simulink model "under_actuated"  (R2020b)
settings: Solver=ode45  StartTime=0.0  StopTime=300  RelTol=1e-3
libraries: simulink x1
settings Model: Creator=kp473  LastModifiedBy=kp473
settings SolverCC: MaxConsecutiveMinStep=10

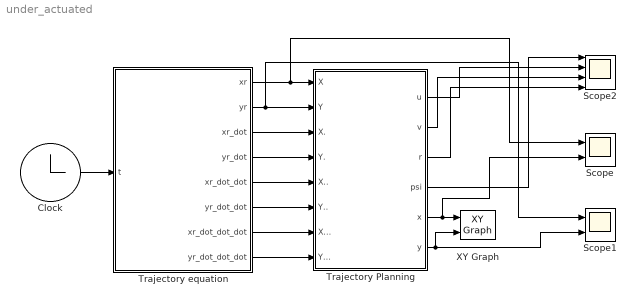
== system under_actuated ==
  Clock : Clock
      settings: Decimation=30
  Scope : Scope  NumInputPorts=2
  Scope1 : Scope  NumInputPorts=2
  Scope2 : Scope  NumInputPorts=4
  Trajectory Planning : Subsystem
  Trajectory equation : MATLAB Function  TreatAsAtomicUnit=on
  XY Graph : simulink/Sinks/XY Graph  xmin=-20  xmax=20  ymin=-20  ymax=20  st=-1
  wires:
  Clock/1 -> Trajectory equation/1(t)
  Trajectory equation/1(xr) -> Scope/1, Trajectory Planning/1(X)
  Trajectory equation/3(xr_dot) -> Trajectory Planning/3(X.)
  Trajectory equation/5(xr_dot_dot) -> Trajectory Planning/5(X..)
  Trajectory equation/2(yr) -> Scope1/1, Trajectory Planning/2(Y)
  Trajectory equation/4(yr_dot) -> Trajectory Planning/4(Y.)
  Trajectory equation/6(yr_dot_dot) -> Trajectory Planning/6(Y..)
  Trajectory equation/7(xr_dot_dot_dot) -> Trajectory Planning/7(X...)
  Trajectory equation/8(yr_dot_dot_dot) -> Trajectory Planning/8(Y...)
  Trajectory Planning/5(x) -> Scope/2, XY Graph/1
  Trajectory Planning/6(y) -> Scope1/2, XY Graph/2
  Trajectory Planning/4(psi) -> Scope2/1
  Trajectory Planning/1(u) -> Scope2/2
  Trajectory Planning/2(v) -> Scope2/3
  Trajectory Planning/3(r) -> Scope2/4

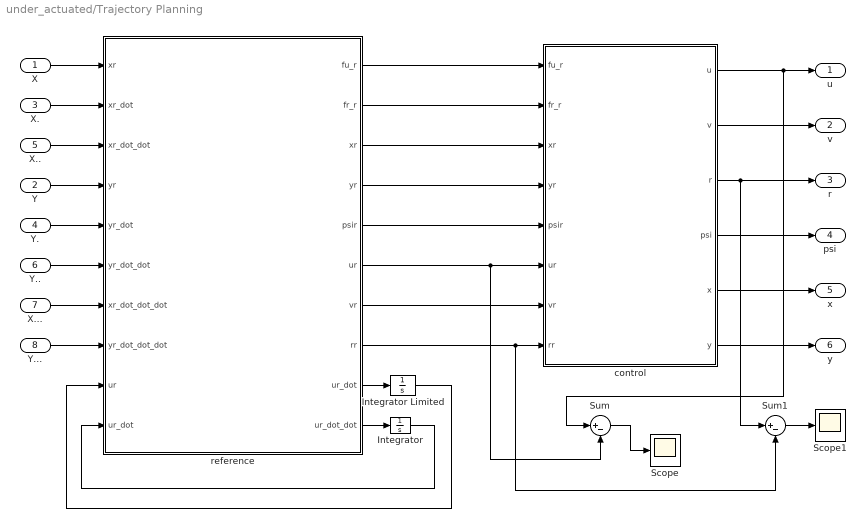
== system under_actuated/Trajectory Planning ==
  X : Inport
  Y : Inport  Port=2
  X. : Inport  Port=3
  Y. : Inport  Port=4
  X.. : Inport  Port=5
  Y.. : Inport  Port=6
  X... : Inport  Port=7
  Y... : Inport  Port=8
  Integrator : Integrator
  Integrator Limited : Integrator  InitialCondition=0.001  LimitOutput=on  UpperSaturationLimit=10  LowerSaturationLimit=-10
  Scope : Scope
  Scope1 : Scope
  Sum : Sum  Inputs=|+-
  Sum1 : Sum  Inputs=|+-
  control : Subsystem
  "reference " : MATLAB Function  TreatAsAtomicUnit=on
  u : Outport
  v : Outport  Port=2
  r : Outport  Port=3
  psi : Outport  Port=4
  x : Outport  Port=5
  y : Outport  Port=6
  wires:
  Y./1 -> "reference "/5(yr_dot)
  X/1 -> "reference "/1("xr ")
  Y../1 -> "reference "/6(yr_dot_dot)
  Y/1 -> "reference "/4("yr ")
  X./1 -> "reference "/2(xr_dot)
  X../1 -> "reference "/3(xr_dot_dot)
  X.../1 -> "reference "/7(xr_dot_dot_dot)
  Y.../1 -> "reference "/8(yr_dot_dot_dot)
  "reference "/10(ur_dot_dot) -> Integrator/1
  Integrator/1 -> "reference "/10("ur_dot ")
  "reference "/9(ur_dot) -> Integrator Limited/1
  Integrator Limited/1 -> "reference "/9("ur ")
  "reference "/1(fu_r) -> control/1(fu_r)
  "reference "/2(fr_r) -> control/2(fr_r)
  "reference "/3(xr) -> control/3(xr)
  "reference "/4(yr) -> control/4(yr)
  "reference "/5(psir) -> control/5(psir)
  "reference "/6(ur) -> Sum/2, control/6(ur)
  "reference "/7(vr) -> control/7(vr)
  "reference "/8(rr) -> Sum1/2, control/8(rr)
  control/1(u) -> Sum/1, u/1
  control/2(v) -> v/1
  control/3(r) -> Sum1/1, r/1
  control/4(psi) -> psi/1
  control/5(x) -> x/1
  control/6(y) -> y/1
  Sum/1 -> Scope/1
  Sum1/1 -> Scope1/1

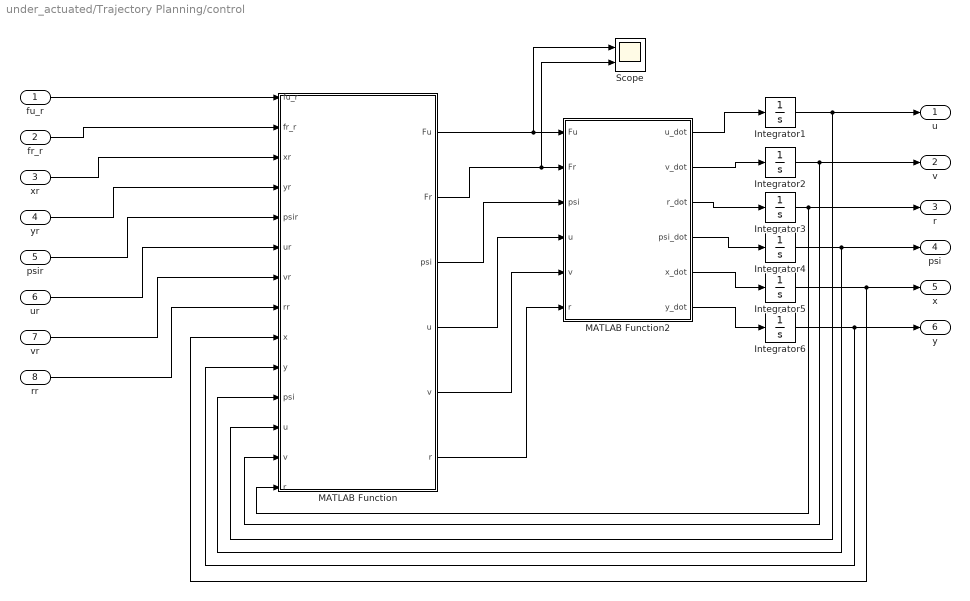
== system under_actuated/Trajectory Planning/control ==
  fu_r : Inport
  fr_r : Inport  Port=2
  xr : Inport  Port=3
  yr : Inport  Port=4
  psir : Inport  Port=5
  ur : Inport  Port=6
  vr : Inport  Port=7
  rr : Inport  Port=8
  Integrator{1..6} (6 alike) : Integrator
  MATLAB Function : MATLAB Function  TreatAsAtomicUnit=on
  MATLAB Function2 : MATLAB Function  TreatAsAtomicUnit=on
  Scope : Scope  NumInputPorts=2
  u : Outport
  v : Outport  Port=2
  r : Outport  Port=3
  psi : Outport  Port=4
  x : Outport  Port=5
  y : Outport  Port=6
  wires:
  Integrator2/1 -> v/1, MATLAB Function/13("v ")
  Integrator3/1 -> r/1, MATLAB Function/14("r ")
  rr/1 -> MATLAB Function/8(rr)
  MATLAB Function/4(u) -> MATLAB Function2/4(u)
  MATLAB Function2/1(u_dot) -> Integrator1/1
  MATLAB Function/2(Fr) -> Scope/2, MATLAB Function2/2(Fr)
  MATLAB Function2/5(x_dot) -> Integrator5/1
  MATLAB Function2/3(r_dot) -> Integrator3/1
  MATLAB Function/6(r) -> MATLAB Function2/6(r)
  Integrator1/1 -> u/1, MATLAB Function/12("u ")
  xr/1 -> MATLAB Function/3(xr)
  MATLAB Function2/2(v_dot) -> Integrator2/1
  Integrator6/1 -> y/1, MATLAB Function/10(y)
  MATLAB Function2/4(psi_dot) -> Integrator4/1
  yr/1 -> MATLAB Function/4(yr)
  Integrator4/1 -> psi/1, MATLAB Function/11("psi ")
  psir/1 -> MATLAB Function/5(psir)
  MATLAB Function/3(psi) -> MATLAB Function2/3(psi)
  MATLAB Function/5(v) -> MATLAB Function2/5(v)
  MATLAB Function/1(Fu) -> Scope/1, MATLAB Function2/1(Fu)
  MATLAB Function2/6(y_dot) -> Integrator6/1
  Integrator5/1 -> x/1, MATLAB Function/9(x)
  fu_r/1 -> MATLAB Function/1(fu_r)
  vr/1 -> MATLAB Function/7(vr)
  fr_r/1 -> MATLAB Function/2(fr_r)
  ur/1 -> MATLAB Function/6(ur)

== matlab function under_actuated/Trajectory equation ==
  data: xr output; yr output; t input; xr_dot output; yr_dot output; xr_dot_dot output; yr_dot_dot output; xr_dot_dot_dot output; yr_dot_dot_dot output
function [xr,yr,xr_dot,yr_dot,xr_dot_dot,yr_dot_dot,xr_dot_dot_dot,yr_dot_dot_dot] = fcn(t)

A = 10;
w = 0.1;

xr = A*sin(w*t);
yr = A*cos(w*t);

xr_dot = A*w*cos(w*t);
yr_dot = -A*w*sin(w*t);

xr_dot_dot = -A*w*w*sin(w*t);
yr_dot_dot = -A*w*w*cos(w*t);

xr_dot_dot_dot= -A*w*w*w*cos(w*t);
yr_dot_dot_dot= A*w*w*w*sin(w*t);

end

== matlab function under_actuated/Trajectory Planning/control/MATLAB Function ==
  data: fu_r input; Fu output; Fr output; fr_r input; xr input; yr input; psir input; ur input; vr input; rr input; x input; y input; psi input; u input; v input; r input; psi output; u output; v output; r output
function [Fu,Fr,psi,u,v,r] = fcn(fu_r, fr_r, xr, yr, psir, ur, vr, rr, x, y, psi, u, v, r)

% constants 
m= 185.0;                                                   % Mass kg
Iz = 50.0;                                                  % Moment of intertia
Xu = -30.0;                                                 
Yv = -90.0;                                                 
Nr = -30.0;                                                 
M = [(m-Xu); (m-Yv); (Iz-Nr)];                              % combined inertia and added mass terms
Minv = [1.0/(m-Xu); 1.0/(m-Yv); 1.0/(Iz-Nr)];               % one by combined inertia and added mass terms
dl = [70.0; 100.0; 50.0];  

% gain and errors
    e_xy = [ x - xr; y - yr];
    e_u = u - ur;
    e_v = v - vr;
    e_r = r - rr;
    e_psi = psi - psir;
    
    R = [ cos(psi), -sin(psi);
            sin(psi), cos(psi)];
    
    cu = 0.5;
    cr = 0.4;
    c = 0.6;
    kc = 0.2;
    
    k = 0.5;
    K = [k, 0;
        0, k];
    
    ku = 0.7;
    k1 = 0.7;
    K1 = [k1, 0;
        0, k1];
       
    alpha_uv = - transpose(R)*(K+K1)*e_xy;
    Zu = e_u - alpha_uv(1);
    Zv = e_v - alpha_uv(2);
    alpha_r = -cr*(-u*Zv*M(1)*Minv(2) + e_psi);
    Zr = e_r - alpha_r;
    
    
% Backstepping Control 
    T_u = -(k+k1)*e_u - cu*Zu - ku*Zu*(k+k1)*(k+k1);    
    T_r = -Zv - e_psi - cr*e_r*(((M(1)*u*Minv(2))^2)+1) - Zr*(c + kc*((cr*M(1)*u*Minv(2))^2));
    
% Updating Input of AUV ( Force and Torque )
    Fu = fu_r + M(1)*T_u + (dl(1)*e_u) - M(2)*(e_v*e_r + e_v*rr + vr*e_r);      
    Fr = fr_r + M(3)*T_r + (dl(3)*e_r) + (M(2)-M(1))*(e_u*e_v+ e_u*vr + ur*e_v);
    
end

== matlab function under_actuated/Trajectory Planning/reference  ==
  data: xr input; xr_dot input; xr_dot_dot input; fu_r output; yr input; yr_dot input; yr_dot_dot input; xr_dot_dot_dot input; yr_dot_dot_dot input; fr_r output; ur input; ur_dot input; xr output; yr output; psir output; ur output; vr output; rr output; ur_dot output; ur_dot_dot output
function [fu_r,fr_r,xr,yr,psir,ur,vr,rr,ur_dot,ur_dot_dot] = fcn(xr, xr_dot, xr_dot_dot,yr,yr_dot, yr_dot_dot,xr_dot_dot_dot,yr_dot_dot_dot,ur,ur_dot)

mass= 185.0;                                                % Mass kg
Iz = 50.0;                                                  % Rotational inertia kg-m2
Xu = -30.0;                                                 % added mass kg
Yv = -90.0;                                                 
Nr = -30.0;                                                 
m = [(mass-Xu); (mass-Yv); (Iz-Nr)];                        % combined inertia and added mass terms
dl = [70.0; 100.0; 50.0];                                    % linear drag 

v_p= sqrt((xr_dot)^2+(yr_dot)^2);
v_p_dot= (xr_dot*xr_dot_dot + yr_dot*yr_dot_dot)/sqrt((xr_dot)^2+(yr_dot)^2);

beta= atan2(yr_dot,xr_dot);
if(beta<0)
            beta = beta + 2*pi;
elseif (beta>6.28)
            beta = beta - 2*pi;
end

omega = ((xr_dot*yr_dot_dot) - (yr_dot*xr_dot_dot))/(v_p^2);

if(omega<=0)    
         if(ur>=0.1)
             ur = 0.1;
             vr = 0;
             rr = 0;
             psir = beta;
                    
         else 
             vr = sqrt((v_p*v_p) - (ur^2));
             gamma = atan2(vr,ur);
             if(gamma<0)
                gamma = gamma + 2*pi;
             elseif (gamma>6.28)
                gamma = gamma - 2*pi;
             end
             psir = beta - gamma;
             rr = omega - ((ur*v_p_dot - ur_dot*v_p)/(v_p*abs(vr)));
         end 
else
         if(ur>=0.1)
             ur = 0.1;
             vr = 0;
             rr = 0;
             psir= beta;
                  
         else
             vr = -sqrt((v_p*v_p) - (ur^2));
             gamma = atan2(vr,ur);
             if(gamma<0)
                gamma = gamma + 2*pi;
             elseif(gamma>6.28)
                 gamma = gamma - 2*pi;
             end
             psir = beta + gamma;
             rr = omega + ((ur*v_p_dot - ur_dot*v_p)/(v_p*abs(vr)));
         end 
end

omega_dot = ((xr_dot*yr_dot_dot_dot) - (yr_dot*xr_dot_dot_dot))/(v_p^2);

if(vr==0)
    ur_dot_dot = 0;
    rr_dot = 0;
    ur_dot = 0;
else 
    ur_dot_dot = -((m(1)*abs(vr)*omega_dot)/(m(1)-m(2))) + ((2*dl(2)*ur_dot)/(m(1)-m(2))) + ((m(1)*omega*(3*ur^2 - v_p^2))/((m(1)-m(2))*ur*abs(vr))) - ((ur_dot^2)/(ur));
    rr_dot = omega_dot - ((v_p*ur_dot_dot)/abs(vr)) + ((v_p*ur*(ur_dot^2))/(abs(vr)*vr*vr));
    ur_dot = ( (dl(2)*v_p*((ur)^2)) - dl(2)*(v_p^3) - (m(1)*omega*ur*v_p*abs(vr)) + (m(1)*ur*ur*v_p_dot) - (m(2)*v_p_dot*v_p*v_p) )/(ur*v_p*(m(1)-m(2)));
end

fu_r = (m(1)*ur_dot)  + (dl(1)*ur) - (m(2)*vr*rr);
fr_r=  (m(3)*rr_dot)  - ((m(2)-m(1))*ur*vr) + (dl(3)*rr) ;


end

== matlab function under_actuated/Trajectory Planning/control/MATLAB Function2 ==
  data: Fu input; u_dot output; Fr input; psi input; v_dot output; r_dot output; psi_dot output; x_dot output; y_dot output; u input; v input; r input
function [u_dot,v_dot,r_dot,psi_dot,x_dot,y_dot] = fcn(Fu,Fr,psi,u,v,r)

m= 185.0;                           % Mass kg
Iz = 50.0;                          % Moment of Inertia
Xu_dot = -30.0;                 
Yv_dot = -90.0;                     
Nr_dot = -30.0;                    
M = [(m-Xu_dot),(m-Yv_dot), (Iz-Nr_dot)];                    % combined inertia and added mass terms
Minv = [1.0/(m-Xu_dot), 1.0/(m-Yv_dot), 1.0/(Iz-Nr_dot)]'; % one by combined inertia and added mass terms
d = [70.0, 100.0, 50.0]';                                    % linear drag [surge, sway, yaw]

u_dot = ((M(2)*v*r)*Minv(1)) + ((-d(1)*u)*Minv(1)) + (Fu*Minv(1));       

v_dot = (-(M(1)*u*r)*Minv(2)) + ((-d(2)*v)*Minv(2));                          

r_dot = (((M(1)-M(2))*u*v)*Minv(3)) + ((-d(3)*r)*Minv(3)) + (Fr*Minv(3)); 

psi_dot = r;                                                                           

x_dot = (u*cos(psi)) - (v*sin(psi));                                           

y_dot = (u*sin(psi)) + (v*cos(psi));
